simulink model "main"  (R2022b)
settings: Solver=VariableStepAuto  StartTime=0.0  StopTime=10.0  RelTol=1e-3
settings Model: Creator=akifa  LastModifiedBy=akifa

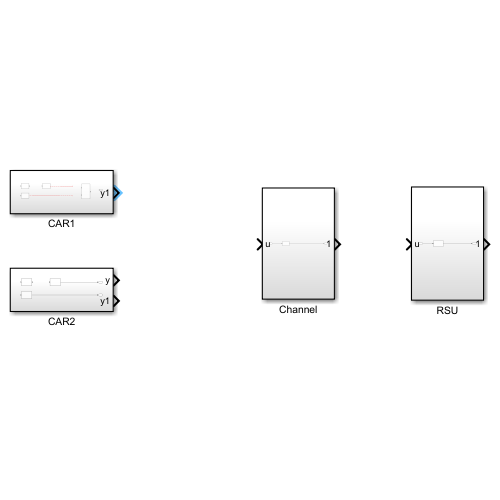
[thumbnail: Simulink's stored preview of the top-level diagram]
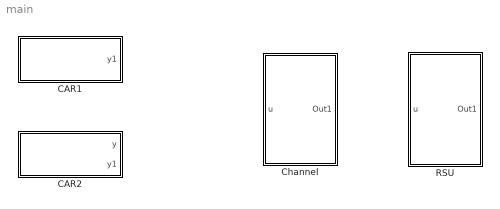
== system main ==
  CAR1 : Subsystem
  CAR2 : Subsystem
  Channel : Subsystem
  RSU : Subsystem

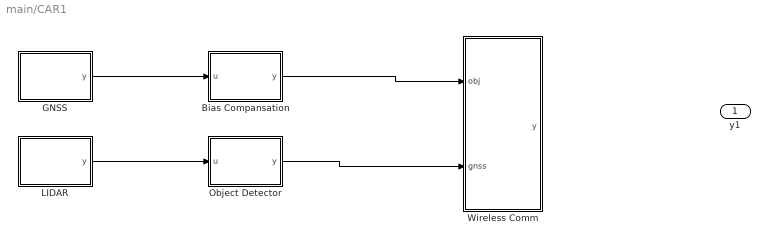
== system main/CAR1 ==
  Bias Compansation : MATLAB Function  TreatAsAtomicUnit=on
  GNSS : MATLAB Function  TreatAsAtomicUnit=on
  LIDAR : MATLAB Function  TreatAsAtomicUnit=on
  Object Detector : MATLAB Function  TreatAsAtomicUnit=on
  Wireless Comm : MATLAB Function  TreatAsAtomicUnit=on
  y1 : Outport
  wires:
  Bias Compansation/1(y) -> Wireless Comm/1(obj)
  LIDAR/1(y) -> Object Detector/1(u)
  GNSS/1(y) -> Bias Compansation/1(u)
  Object Detector/1(y) -> Wireless Comm/2(gnss)

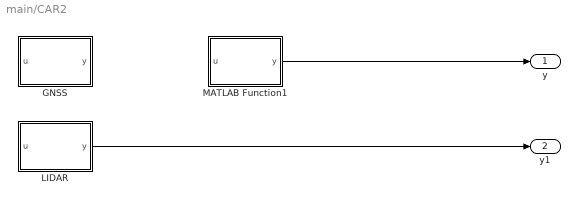
== system main/CAR2 ==
  GNSS : MATLAB Function  TreatAsAtomicUnit=on
  LIDAR : MATLAB Function  TreatAsAtomicUnit=on
  MATLAB Function1 : MATLAB Function  TreatAsAtomicUnit=on
  y : Outport
  y1 : Outport  Port=2
  wires:
  MATLAB Function1/1(y) -> y/1
  LIDAR/1(y) -> y1/1

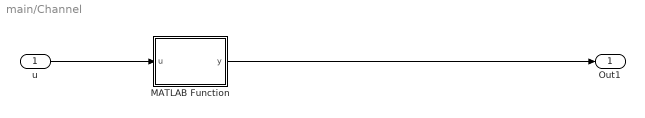
== system main/Channel ==
  u : Inport
  MATLAB Function : MATLAB Function  TreatAsAtomicUnit=on
  Out1 : Outport
  wires:
  MATLAB Function/1(y) -> Out1/1
  u/1 -> MATLAB Function/1(u)

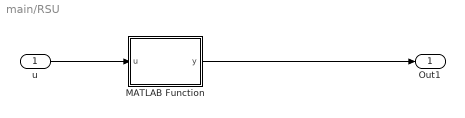
== system main/RSU ==
  u : Inport
  MATLAB Function : MATLAB Function  TreatAsAtomicUnit=on
  Out1 : Outport
  wires:
  MATLAB Function/1(y) -> Out1/1
  u/1 -> MATLAB Function/1(u)

== matlab function main/CAR1/GNSS ==
  data: y output
function y = fcn()

y = u;

== matlab function main/Channel/MATLAB Function ==
  data: u input; y output
function y = fcn(u)

y = u;

== matlab function main/RSU/MATLAB Function ==
  data: u input; y output
function y = fcn(u)

y = u;

== matlab function main/CAR1/Bias Compansation ==
  data: u input; y output
function y = fcn(u)

y = u;

== matlab function main/CAR1/LIDAR ==
  data: y output
function y = fcn()

y = u;

== matlab function main/CAR2/LIDAR ==
  data: u input; y output
function y = fcn(u)

y = u;

== matlab function main/CAR2/MATLAB Function1 ==
  data: u input; y output
function y = fcn(u)

y = u;

== matlab function main/CAR1/Wireless Comm ==
  data: obj input; y output; gnss input
function y = fcn(obj, gnss)

y = u;

== matlab function main/CAR1/Object Detector ==
  data: u input; y output
function y = fcn(u)

y = u;

== matlab function main/CAR2/GNSS ==
  data: u input; y output
function y = fcn(u)

y = u;
